simulink model "lab_7_sldemo_bounce"  (R2018a)
settings: Solver=ode23  StartTime=0.0  StopTime=time_s*3  MaxStep=0.01  RelTol=1e-3  AbsTol=1E-6  EnableMultiTasking=on
values from neighbouring files (symbols this model uses):
  drag3 = calculate_drag_f(drag_coef, air_rho, metal_ball_M_kg, metal_ball_R_m)    [constants_lab7.m]
  V_0_Y = sind(angle_d) * V_0    [constants_lab7.m]
libraries: simulink x1
Description:
  | Bouncing Ball Model
  | 
  | This model calculates the trajectory, over time, of a ball thrown
  | upward with a velocity of 15 meters per second from a height of 10 m.
  | The model demonstrates the use of the 'ReinitDXDTwhenXreachesSaturation'
  | parameter in the Second-Order Integrator block to model this system.
  | This parameter, when set to 'on', forces a reinitialization of dx/dt
  | (velocity in the model) at the instant when x (position) reaches
  | saturation (i.e., when the ball hits the ground). The reinitialized value
  | is calculated by multiplying a coefficient of restitution times the ball
  | velocity, the instant before the ball hits the ground. The Memory block
  | in the calculation loop serves to capture the velocity of the ball just
  | before it hits the ground. The position of the ball is plotted in the
  | upper axis of the scope while the velocity of the ball is plotted in
  | the lower axis.
settings Model: Creator=The MathWorks, Inc.  LastModifiedBy=user
settings SolverCC: AutoScaleAbsTol=off
settings DataIOCC: MaxDataPoints=7500  SaveFormat=Array  SaveOutput=off  SignalLogging=off  DSMLogging=off  SaveTime=off
settings OptimizationCC: ExpressionDepthLimit=2147483647  EfficientFloat2IntCast=on  LifeSpan=inf
settings DebuggingCC: UnderspecifiedInitializationDetection=Classic  MergeDetectMultiDrivingBlocksExec=none  IgnoredZcDiagnostic=none  FcnCallInpInsideContextMsg=warning  StateNameClashWarn=warning  SFUnexpectedBacktrackingDiag=warning  SFNoUnconditionalDefaultTransitionDiag=warning  SFExecutionAtInitializationDiag=none
settings HardwareCC: ProdBitPerPointer=32  ProdBitPerSizeT=32  ProdBitPerPtrDiffT=32  ProdLargestAtomicFloat=None  ProdIntDivRoundTo=Undefined  ProdEndianess=Unspecified  ProdWordSize=32  ProdHWDeviceType=32-bit Generic  TargetBitPerPointer=64  TargetBitPerSizeT=64  TargetBitPerPtrDiffT=64  TargetLongLongMode=on  TargetIntDivRoundTo=Zero  TargetEndianess=LittleEndian  TargetWordSize=64  TargetHWDeviceType=MATLAB Host  ProdEqTarget=off
settings ModelReferenceCC: PropagateSignalLabelsOutOfModel=off
settings RTWCC: SystemTargetFile=rsim.tlc  TemplateMakefile=rsim_default_tmf  Description=Rapid Simulation Target
settings CodeAppCC: StateflowObjectComments=on
settings ConfigComp: CovMetricSettings=dw  CovHtmlReporting=on  CovSaveCumulativeToWorkspaceVar=on  CovSaveSingleToWorkspaceVar=on  CovExternalEMLEnable=off

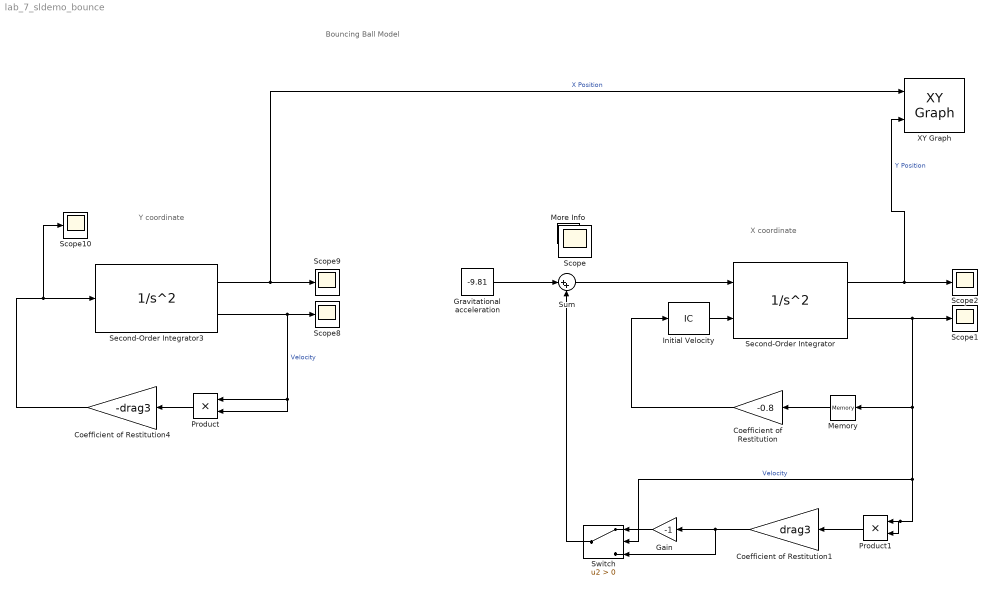
== system lab_7_sldemo_bounce ==
  note: Bouncing Ball Model
  note: Y coordinate
  note: X coordinate
  Coefficient of Restitution : Gain  Gain=-0.8
  Coefficient of Restitution1 : Gain  Gain=drag3
  Coefficient of Restitution4 : Gain  Gain=-drag3
  Gain : Gain  Gain=-1
  Gravitational acceleration : Constant  Value=-9.81  OutDataTypeStr=double
  "Initial Velocity " : InitialCondition  Value=V_0_Y
  Memory : Memory
  More Info : Subsystem
      settings: OpenFcn=showExample('simulink_general/sldemo_bounceExample')
      mask Display: disp('?')
  Product : Product
  Product1 : Product
  Scope{,1..2,8..10} (6 alike) : Scope
  Second-Order Integrator : SecondOrderIntegrator  ICX=H_0  LimitX=on  LowerLimitX=0.0  StateNameX='Position'  ICSourceDXDT=external  StateNameDXDT='Velocity'  ReinitDXDTwhenXreachesSaturation=on
  Second-Order Integrator3 : SecondOrderIntegrator  ICX=0  LimitX=on  LowerLimitX=0.0  StateNameX='Position'  ICDXDT=V_0_X  StateNameDXDT='Velocity'  ReinitDXDTwhenXreachesSaturation=on
  Sum : Sum  Inputs=|++
  Switch : Switch  Criteria=u2 > Threshold
  XY Graph : simulink/Sinks/XY Graph  xmin=0  xmax=120  ymin=0  ymax=35  st=-1
  wires:
  Second-Order Integrator/1 -> XY Graph/2, Scope2/1  "Y Position"
  Second-Order Integrator/2 -> Scope1/1, Switch/2, Product1/2, Product1/1, Memory/1  "Velocity"
  Memory/1 -> Coefficient of Restitution/1
  "Initial Velocity "/1 -> Second-Order Integrator/2
  Coefficient of Restitution/1 -> "Initial Velocity "/1
  Product/1 -> Coefficient of Restitution4/1
  Second-Order Integrator3/2 -> Product/2, Product/1, Scope8/1  "Velocity"
  Second-Order Integrator3/1 -> XY Graph/1, Scope9/1  "X Position"
  Coefficient of Restitution4/1 -> Second-Order Integrator3/1, Scope10/1
  Product1/1 -> Coefficient of Restitution1/1
  Gain/1 -> Switch/1
  Coefficient of Restitution1/1 -> Switch/3, Gain/1
  Switch/1 -> Sum/2
  Sum/1 -> Second-Order Integrator/1
  Gravitational acceleration/1 -> Sum/1

== system lab_7_sldemo_bounce/More Info ==
